simulink model "DIsc2"  (R2020a)
settings: Solver=ode45  StartTime=0.0  StopTime=5e-4  RelTol=1e-6  AbsTol=1e-6
InitFcn:
  | R1 = 1000;
  | R2 = 20;
  | L = 25.3E-6;
  | C = 100E-9;
  | Is = 1E-8;
  | UT = 26E-3;
  | f = 0.15E+6;
model workspace (MAT data in the model file):
  C = 1e-07
  L = 2.53e-05
  R1 = 1000
  R2 = 20
  f = 150000
settings Model: Creator=Lisa  LastModifiedBy=peter
settings DataIOCC: ReturnWorkspaceOutputs=off  OutputOption=SpecifiedOutputTimes  OutputTimes=0:1e-8:5e-4

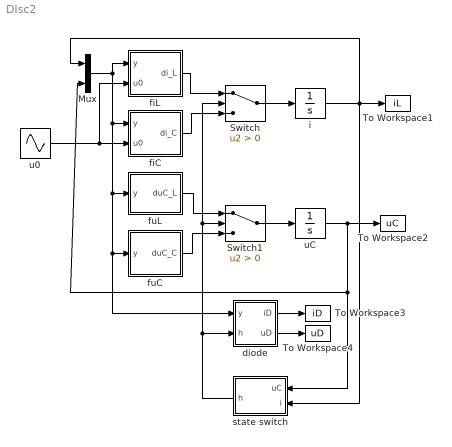
== system DIsc2 ==
  Mux : Mux  Inputs=2
  Switch : Switch  Criteria=u2 > Threshold
  Switch1 : Switch  Criteria=u2 > Threshold
  To Workspace1 : ToWorkspace  VariableName=iL  SaveFormat=Timeseries  SampleTime=-1
  To Workspace2 : ToWorkspace  VariableName=uC  SaveFormat=Timeseries  SampleTime=-1
  To Workspace3 : ToWorkspace  VariableName=iD  SaveFormat=Timeseries  SampleTime=-1
  To Workspace4 : ToWorkspace  VariableName=uD  SaveFormat=Timeseries  SampleTime=-1
  diode : Subsystem
  fiC : Subsystem
  "fiL " : Subsystem
  fuC : Subsystem
  fuL : Subsystem
  i : Integrator
  state switch : Subsystem
  u0 : Sin  Amplitude=-1  Frequency=2*pi*f  SampleTime=0
  uC : Integrator
  wires:
  Switch/1 -> i/1
  Switch1/1 -> uC/1
  "fiL "/1(di_L) -> Switch/1
  fuL/1(duC_L) -> Switch1/1
  fuC/1(duC_C) -> Switch1/3
  fiC/1(di_C) -> Switch/3
  state switch/1(h) -> diode/2(h), Switch/2, Switch1/2
  i/1 -> To Workspace1/1, Mux/1, state switch/2(i)
  Mux/1 -> diode/1(y), fuC/1(y), fuL/1(y), fiC/1(y), "fiL "/1(y)
  uC/1 -> state switch/1(uC), Mux/2, To Workspace2/1
  u0/1 -> "fiL "/2(u0), fiC/2(u0)
  diode/1(iD) -> To Workspace3/1
  diode/2(uD) -> To Workspace4/1

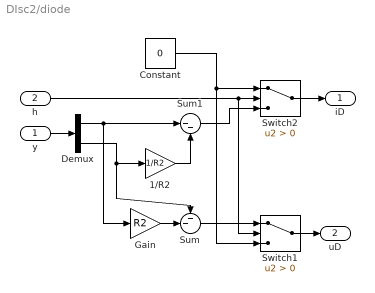
== system DIsc2/diode ==
  y : Inport
  h : Inport  Port=2
  1/R2 : Gain  Gain=1/R2
  Constant : Constant  Value=0
  Demux : Demux  Outputs=2
  Gain : Gain  Gain=R2
  Sum : Sum  Inputs=--|
  Sum1 : Sum  Inputs=|--
  Switch1 : Switch  Criteria=u2 > Threshold
  Switch2 : Switch  Criteria=u2 > Threshold
  iD : Outport
  uD : Outport  Port=2
  wires:
  y/1 -> Demux/1
  h/1 -> Switch1/2, Switch2/2
  Switch1/1 -> uD/1
  Switch2/1 -> iD/1
  Demux/1 -> Gain/1, Sum1/1
  Demux/2 -> 1/R2/1, Sum/1
  Constant/1 -> Switch1/3, Switch2/1
  Sum/1 -> Switch1/1
  Gain/1 -> Sum/2
  Sum1/1 -> Switch2/3
  1/R2/1 -> Sum1/2

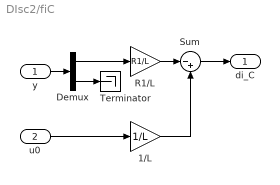
== system DIsc2/fiC ==
  y : Inport
  u0 : Inport  Port=2
  1/L : Gain  Gain=1/L
  Demux : Demux  Outputs=2
  R1/L : Gain  Gain=R1/L
  Sum : Sum  Inputs=|-+
  Terminator : Terminator
  di_C : Outport
  wires:
  y/1 -> Demux/1
  u0/1 -> 1/L/1
  Sum/1 -> di_C/1
  Demux/1 -> R1/L/1
  R1/L/1 -> Sum/1
  Demux/2 -> Terminator/1
  1/L/1 -> Sum/2

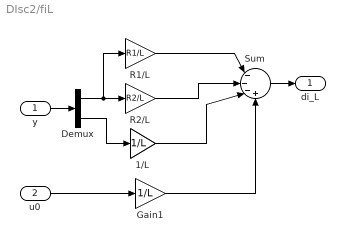
== system DIsc2/fiL  ==
  y : Inport
  u0 : Inport  Port=2
  1/L : Gain  Gain=1/L
  Demux : Demux  Outputs=2
  Gain1 : Gain  Gain=1/L
  R1/L : Gain  Gain=R1/L
  R2/L : Gain  Gain=R2/L
  Sum : Sum  Inputs=|---+
  di_L : Outport
  wires:
  y/1 -> Demux/1
  Demux/2 -> 1/L/1
  Sum/1 -> di_L/1
  R1/L/1 -> Sum/1
  Demux/1 -> R1/L/1, R2/L/1
  R2/L/1 -> Sum/2
  1/L/1 -> Sum/3
  u0/1 -> Gain1/1
  Gain1/1 -> Sum/4

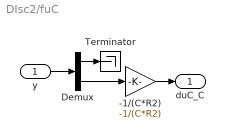
== system DIsc2/fuC ==
  y : Inport
  -1/(C*R2) : Gain  Gain=-1/(C*R2)
  Demux : Demux  Outputs=2
  Terminator : Terminator
  duC_C : Outport
  wires:
  y/1 -> Demux/1
  Demux/2 -> -1/(C*R2)/1
  -1/(C*R2)/1 -> duC_C/1
  Demux/1 -> Terminator/1

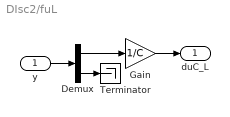
== system DIsc2/fuL ==
  y : Inport
  Demux : Demux  Outputs=2
  Gain : Gain  Gain=1/C
  Terminator : Terminator
  duC_L : Outport
  wires:
  y/1 -> Demux/1
  Demux/1 -> Gain/1
  Gain/1 -> duC_L/1
  Demux/2 -> Terminator/1

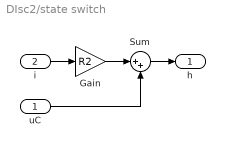
== system DIsc2/state switch ==
  uC : Inport
  i : Inport  Port=2
  Gain : Gain  Gain=R2
  Sum : Sum  Inputs=|++
  h : Outport
  wires:
  Gain/1 -> Sum/1
  i/1 -> Gain/1
  uC/1 -> Sum/2
  Sum/1 -> h/1
